simulink model "q_1_10"  (R2020a)
settings: Solver=VariableStepAuto  StartTime=0.0  StopTime=60  RelTol=1e-3
libraries: simulink x1
settings Model: Creator=debora  LastModifiedBy=dimit

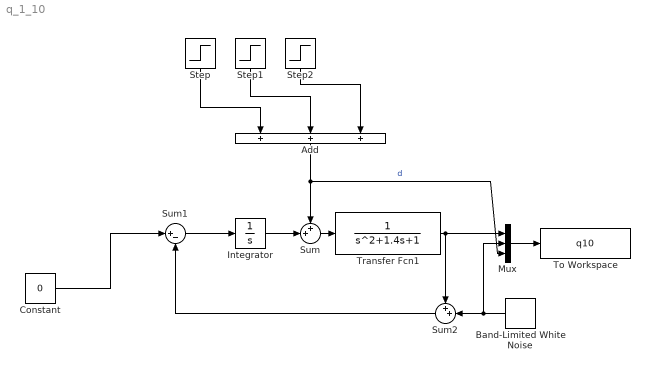
== system q_1_10 ==
  Add : Sum  Inputs=3
  Band-Limited White Noise : simulink/Sources/Band-Limited White Noise  Cov=[0.01]  Ts=0.1  seed=[23341]
  Constant : Constant  Value=0
  Integrator : Integrator
  Mux : Mux  Inputs=3
  Step : Step  Time=0  After=-1  SampleTime=0
  Step1 : Step  Time=6  After=3  SampleTime=0
  Step2 : Step  Time=15  After=-1  SampleTime=0
  Sum : Sum  Inputs=++|
  Sum1 : Sum  Inputs=|+-
  Sum2 : Sum  Inputs=++|
  To Workspace : ToWorkspace  VariableName=q10  SaveFormat=Timeseries  SampleTime=-1
  Transfer Fcn1 : TransferFcn  Denominator=[1 1.4 1]
  wires:
  Integrator/1 -> Sum/2
  Step1/1 -> Add/2
  Step2/1 -> Add/3
  Add/1 -> Mux/3, Sum/1  "d"
  Sum1/1 -> Integrator/1
  Sum2/1 -> Sum1/2
  Band-Limited White Noise/1 -> Mux/2, Sum2/2
  Mux/1 -> To Workspace/1
  Step/1 -> Add/1
  Constant/1 -> Sum1/1
  Sum/1 -> Transfer Fcn1/1
  Transfer Fcn1/1 -> Mux/1, Sum2/1
